simulink model "drone_simul10"  (R2022b)
settings: Solver=VariableStepAuto  StartTime=0.0  StopTime=10  RelTol=1e-3
model workspace (MAT data in the model file):
  Pmax = Simulink.Parameter
  Pmax.Value = 2
  Pmax.DataType = 'auto'
  Pmax.Complexity = 'real'
  Pmax.Dimensions = [1 1]
  g = Simulink.Parameter
  g.Value = 9.81
  g.DataType = 'auto'
  g.Complexity = 'real'
  g.Dimensions = [1 1]
libraries: slpidlib x4, aerolibanimutils x2
settings Model: Creator=Raphael  LastModifiedBy=Raphael
settings OptimizationCC: DefaultParameterBehavior=Inlined  UseDivisionForNetSlopeComputation=on  GainParamInheritBuiltInType=on  UseFloatMulNetSlope=on  InlineInvariantSignals=on  EnhancedBackFolding=on  BooleansAsBitfields=on  PassReuseOutputArgsAs=Individual arguments  StateBitsets=on  DataBitsets=on  ZeroExternalMemoryAtStartup=off  ZeroInternalMemoryAtStartup=off  NoFixptDivByZeroProtection=on  EfficientFloat2IntCast=on  LifeSpan=1  OptimizeBlockOrder=speed  DifferentSizesBufferReuse=on  EfficientTunableParamExpr=on
settings DebuggingCC: ParameterTunabilityLossMsg=error
settings HardwareCC: ProdBitPerLong=64  ProdHWDeviceType=AMD->x86-64 (Linux 64)
settings SFSimCC: MATLABDynamicMemAlloc=off
settings RTWCC: Description=Embedded Coder  SystemTargetFile=ert.tlc  GenCodeOnly=on  TemplateMakefile=ert_default_tmf
settings CodeAppCC: ForceParamTrailComments=on  IgnoreCustomStorageClasses=off  OperatorAnnotations=on  SimulinkDataObjDesc=on  SFDataObjDesc=on  CustomSymbolStrGlobalVar=rt$N$M  CustomSymbolStrType=$N$M  CustomSymbolStrFcn=$N$M$F  CustomSymbolStrMacro=$N$M  InsertBlockDesc=on
settings ERTTargetCC: TargetLangStandard=C99 (ISO)  GenerateSampleERTMain=on  IncludeMdlTerminateFcn=off  CombineSignalStateStructs=on  SupportAbsoluteTime=off  SupportComplex=off  SupportNonInlinedSFcns=on  InlinedParameterPlacement=NonHierarchical  ERTCustomFileTemplate=example_file_process.tlc  ERTFilePackagingFormat=CompactWithDataFile

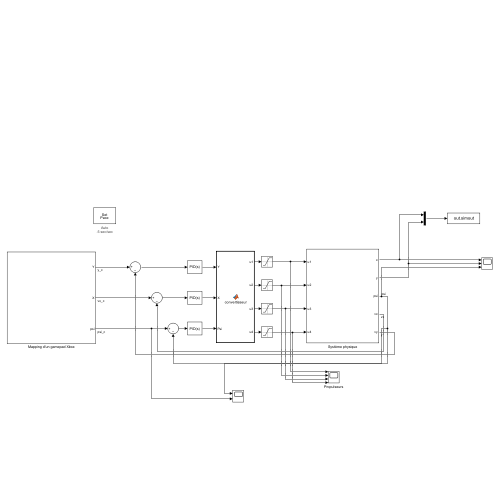
[thumbnail: Simulink's stored preview of the top-level diagram]
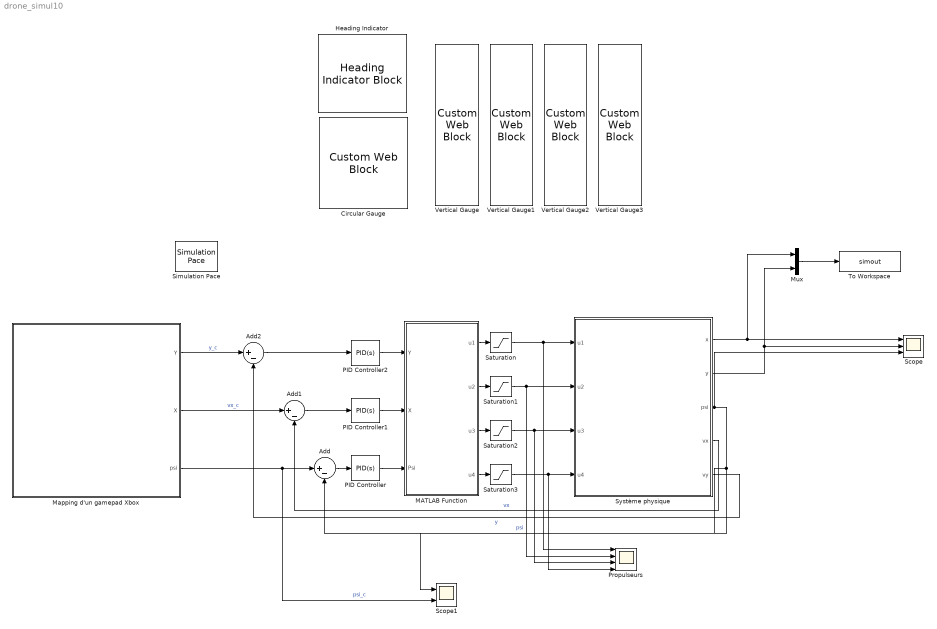
== system drone_simul10 ==
  Add : Sum  Inputs=|+-
  Add1 : Sum  Inputs=|+-
  Add2 : Sum  Inputs=|+-
  Circular Gauge : CustomWebBlock  LabelPosition=Hide  ShowInitialText=on  Configuration="{\"type\":\"CircularGauge\",\"settings\":{\"BindingType\":\"signal\",\"aspectRatio\":1.032258064516129,\"backgroundColor\":[0,0,0,\"1\"],\"backgroundOffset\":1,\"backgroundOpacity\":1,\"direction\":\"cw\",\"fixedAspectRatio\":\"on\",\"flipLimits\":0,\"orientation\":\"horizontal\",\"showBackgroundColor\":false,\"value\":0},\"components\":[{\"name\":\"CircularScaleComponent\",\"settings\":{\"bounds\":{\"max\":10,\"min\":-10,\"tickInterval\":\"auto\"},\"direction\":\"cw\",\"flipLimits\":0,\"innerRadius\":0.75,\"internalTickHeightScaleFactor\":1,\"labelColor\":[255,255,200],\"labelFont\":{\"font\":\"Arial\",\"fontSize\":12},\"labelRadius\":0.528,\"labelTransparency\":1,\"minorTickHeightScaleFactor\":0.2,\"needleImage\":{\"size\":[200,50],\"src\":\"data:image/svg+xml;base64,PD94bWwgdmVyc2lvbj0iMS4wIiBlbmNvZGluZz0idXRmLTgiPz4KPCEtLSBHZW5lcmF0b3I6IEFkb2JlIElsbHVzdHJhdG9yIDI0LjEuMiwgU1ZHIEV4cG9ydCBQbHVnLUluIC4gU1ZHIFZlcnNpb246IDYuMDAgQnVpbGQgMCkgIC0tPgo8c3ZnIHZlcnNpb249IjEuMSIgaWQ9IkxheWVyXzEiIHhtbG5zPSJodHRwOi8vd3d3LnczLm9yZy8yMDAwL3N2ZyIgeG1sbnM6eGxpbms9Imh0dHA6Ly93d3cudzMub3JnLzE5OTkveGxpbmsiIHg9IjBweCIgeT0iMHB4IgoJIHZpZXdCb3g9IjAgMCAyMDAgNTAiIHN0eWxlPSJlbmFibGUtYmFja2dyb3VuZDpuZXcgMCAwIDIwMCA1MDsiIHhtbDpzcGFjZT0icHJlc2VydmUiPgo8c3R5bGUgdHlwZT0idGV4dC9jc3MiPgoJLnN0MHtmaWxsOiNFQzIxMjc7fQo8L3N0eWxlPgo8cGF0aCBjbGFzcz0ic3QwIiBkPSJNMTYyLjgsMTMuN0MxNjksNC40LDE4MS43LDEuOSwxOTEsOC4xczExLjgsMTguOSw1LjYsMjguMnMtMTguOSwxMS44LTI4LjIsNS42bDAsMAoJQzE1OS4xLDM1LjYsMTU2LjYsMjMsMTYyLjgsMTMuN0wxNjIuOCwxMy43eiBNMTY1LjgsMTUuOGMtNS4xLDcuNi0zLjEsMTcuOSw0LjYsMjNjNy42LDUuMSwxNy45LDMuMSwyMy00LjYKCWM1LjEtNy42LDMuMS0xNy45LTQuNi0yM2wwLDBDMTgxLjIsNi4yLDE3MC45LDguMiwxNjUuOCwxNS44eiIvPgo8cGF0aCBjbGFzcz0ic3QwIiBkPSJNMC40LDI1Ljl2LTMuM2wxNTktMi41Yy0wLjcsMi42LTAuNyw1LjIsMCw3LjhMMC40LDI1Ljl6Ii8+CjxjaXJjbGUgY2xhc3M9InN0MCIgY3g9IjE3OS42IiBjeT0iMjQiIHI9IjAuNyIvPgo8L3N2Zz4K\"},\"needleOffset\":[0.18464878250906522,0],\"needleOrientation\":-45,\"needleRotation\":180,\"needleSize\":{\"height\":0.11741692305346914,\"width\":0.46108337545091255},\"outerRadius\":0.9,\"position\":[0.05,0.05,0.9,0.9],\"referencePoint\":\"auto\",\"scaleAngle\":270,\"scaleAngleOffset\":135,\"scaleColors\":[],\"scaleColorsSize\":0.2,\"scaleDirection\":\"CW\",\"scalePosition\":[0,0,1,1],\"showLabels\":1,\"showMinorTicks\":1,\"showSpanLine\":1,\"showTicks\":1,\"tickColor\":[252,252,197],\"tickTransparency\":1,\"valueBarColor\":[0,114,189],\"valueBarPosition\":[0,0,1,1],\"valueBarSize\":0.2,\"valueBarTransparency\":1}},{\"name\":\"BackgroundImageComponent\",\"settings\":{\"image\":{\"size\":[500,500],\"src\":\"data:image/svg+xml;base64,PD94bWwgdmVyc2lvbj0iMS4wIiBlbmNvZGluZz0iVVRGLTgiIHN0YW5kYWxvbmU9Im5vIj8+CjxzdmcKICAgeG1sbnM6ZGM9Imh0dHA6Ly9wdXJsLm9yZy9kYy9lbGVtZW50cy8xLjEvIgogICB4bWxuczpjYz0iaHR0cDovL2NyZWF0aXZlY29tbW9ucy5vcmcvbnMjIgogICB4bWxuczpyZGY9Imh0dHA6Ly93d3cudzMub3JnLzE5OTkvMDIvMjItcmRmLXN5bnRheC1ucyMiCiAgIHhtbG5zOnN2Zz0iaHR0cDovL3d3dy53My5vcmcvMjAwMC9zdmciCiAgIHhtbG5zPSJodHRwOi8vd3d3LnczLm9yZy8yMDAwL3N2ZyIKICAgeG1sbnM6 ...(+9964 chars)\"},\"position\":[0,0,1,1],\"scaleMode\":\"0\"}},{\"name\":\"ForegroundImageComponent\",\"settings\":{\"image\":{\"size\":[0,0],\"src\":\"default\",\"srcOrientation\":[]},\"isForeground\":1,\"position\":[0,0,1,1],\"scaleMode\":\"0\"}}]}"
  Heading Indicator : HeadingIndicatorBlock
  MATLAB Function : MATLAB Function  TreatAsAtomicUnit=on
  Mapping d'un gamepad Xbox : Subsystem
  Mux : Mux  Inputs=2
  PID Controller : slpidlib/PID Controller  Controller=PID  Form=Ideal  TimeDomain=Continuous-time  UseExternalTs=off  SampleTime=-1  IntegratorMethod=Forward Euler  FilterMethod=Forward Euler  ControllerParametersSource=internal  P=5  I=0  UseKiTs=off  D=0.04  N=100  UseFilter=on  TunerSelectOption=Transfer Function Based (PID Tuner App)  InitialConditionSource=internal  InitialConditionForIntegrator=0  InitialConditionForFilter=0  DifferentiatorICPrevScaledInput=0  ExternalReset=none  TrackingMode=off  Kt=1  LimitOutput=off  SatLimitsSource=internal  UpperSaturationLimit=inf  LowerSaturationLimit=-inf  LinearizeAsGain=on  AntiWindupMode=none  Kb=1  LimitIntegrator=off  UpperIntegratorSaturationLimit=inf  LowerIntegratorSaturationLimit=-inf  POutMin=[]  POutMax=[]  IOutMin=[]  IOutMax=[]  DOutMin=[]  DOutMax=[]  NOutMin=[]  NOutMax=[]  SumOutMin=[]  SumOutMax=[]  SaturationOutMin=[]  SaturationOutMax=[]  PParamMin=[]  PParamMax=[]  IParamMin=[]  IParamMax=[]  DParamMin=[]  DParamMax=[]  NParamMin=[]  NParamMax=[]  KbParamMin=[]  KbParamMax=[]  KtParamMin=[]  KtParamMax=[]  KbOutMin=[]  KbOutMax=[]  KtOutMin=[]  KtOutMax=[]  IntegratorOutMin=[]  IntegratorOutMax=[]  FilterOutMin=[]  FilterOutMax=[]  SumI1OutMin=[]  SumI1OutMax=[]  SumI2OutMin=[]  SumI2OutMax=[]  SumI3OutMin=[]  SumI3OutMax=[]  SumI4OutMin=[]  SumI4OutMax=[]  SumDOutMin=[]  SumDOutMax=[]  DifferentiatorOutMin=[]  DifferentiatorOutMax=[]  FilterDiffOutCoefMin=[]  FilterDiffOutCoefMax=[]  ReciprocalOutMin=[]  ReciprocalOutMax=[]  SumDenOutMin=[]  SumDenOutMax=[]  SumNumOutMin=[]  SumNumOutMax=[]  DivideOutMin=[]  DivideOutMax=[]  UdiffTsProdOutMin=[]  UdiffTsProdOutMax=[]  NTsProdOutMin=[]  NTsProdOutMax=[]  UintegralTsProdOutMin=[]  UintegralTsProdOutMax=[]  UngainTsProdOutMin=[]  UngainTsProdOutMax=[]  ClampingZeroOutDataTypeStr=Inherit: Inherit via back propagation  ClampingZeroOutMin=[]  ClampingZeroOutMax=[]  FilterDenConstantOutDataTypeStr=Inherit: Inherit via back propagation  FilterDenConstantOutMin=[]  FilterDenConstantOutMax=[]  PCopyOutDataTypeStr=Inherit: Inherit via back propagation  PCopyOutMin=[]  PCopyOutMax=[]  NCopyOutDataTypeStr=Inherit: Inherit via back propagation  NCopyOutMin=[]  NCopyOutMax=[]  IntegratorContinuousStateAttributes=''  IntegratorStateMustResolveToSignalObject=off  IntegratorRTWStateStorageClass=Auto  FilterContinuousStateAttributes=''  FilterStateMustResolveToSignalObject=off  FilterRTWStateStorageClass=Auto  ParallelPVariant=Passthrough  IdealPVariant=InternalParameters  IVariant=InternalParameters  DVariant=InternalParameters  IntegratorVariant=Continuous  SatVariant=Disabled  AWVariant=Passthrough  PCopyVariant=Disabled  TRVariant=Disabled  FdbkBlocksVariant=Forward  IdealPFdbkVariant=Disabled  SatFdbkVariant=Disabled  DerivativeFilterVariant=ContFilter  NVariant=InternalParameters  NCopyVariant=Disabled  FilterICVariant=InternalICsFilter  IntegratorICVariant=InternalICs  ExternalResetVariant=Disabled  TRSumVariant=Passthrough  SumFdbkVariant=Disabled  SumVariant=Sum_PID  TsampFilterVariant=InternalTs  TsampNgainVariant=Passthrough  TsampIntegralVariant=Passthrough  ExternalSaturationOutDataTypeStr=Inherit: Same as second input
  PID Controller1 : slpidlib/PID Controller  Controller=PID  Form=Ideal  TimeDomain=Continuous-time  UseExternalTs=off  SampleTime=-1  IntegratorMethod=Forward Euler  FilterMethod=Forward Euler  ControllerParametersSource=internal  P=5  I=0.1  UseKiTs=off  D=0  N=100  UseFilter=on  TunerSelectOption=Transfer Function Based (PID Tuner App)  InitialConditionSource=internal  InitialConditionForIntegrator=0  InitialConditionForFilter=0  DifferentiatorICPrevScaledInput=0  ExternalReset=none  TrackingMode=off  Kt=1  LimitOutput=off  SatLimitsSource=internal  UpperSaturationLimit=inf  LowerSaturationLimit=-inf  LinearizeAsGain=on  AntiWindupMode=none  Kb=1  LimitIntegrator=off  UpperIntegratorSaturationLimit=inf  LowerIntegratorSaturationLimit=-inf  POutMin=[]  POutMax=[]  IOutMin=[]  IOutMax=[]  DOutMin=[]  DOutMax=[]  NOutMin=[]  NOutMax=[]  SumOutMin=[]  SumOutMax=[]  SaturationOutMin=[]  SaturationOutMax=[]  PParamMin=[]  PParamMax=[]  IParamMin=[]  IParamMax=[]  DParamMin=[]  DParamMax=[]  NParamMin=[]  NParamMax=[]  KbParamMin=[]  KbParamMax=[]  KtParamMin=[]  KtParamMax=[]  KbOutMin=[]  KbOutMax=[]  KtOutMin=[]  KtOutMax=[]  IntegratorOutMin=[]  IntegratorOutMax=[]  FilterOutMin=[]  FilterOutMax=[]  SumI1OutMin=[]  SumI1OutMax=[]  SumI2OutMin=[]  SumI2OutMax=[]  SumI3OutMin=[]  SumI3OutMax=[]  SumI4OutMin=[]  SumI4OutMax=[]  SumDOutMin=[]  SumDOutMax=[]  DifferentiatorOutMin=[]  DifferentiatorOutMax=[]  FilterDiffOutCoefMin=[]  FilterDiffOutCoefMax=[]  ReciprocalOutMin=[]  ReciprocalOutMax=[]  SumDenOutMin=[]  SumDenOutMax=[]  SumNumOutMin=[]  SumNumOutMax=[]  DivideOutMin=[]  DivideOutMax=[]  UdiffTsProdOutMin=[]  UdiffTsProdOutMax=[]  NTsProdOutMin=[]  NTsProdOutMax=[]  UintegralTsProdOutMin=[]  UintegralTsProdOutMax=[]  UngainTsProdOutMin=[]  UngainTsProdOutMax=[]  ClampingZeroOutDataTypeStr=Inherit: Inherit via back propagation  ClampingZeroOutMin=[]  ClampingZeroOutMax=[]  FilterDenConstantOutDataTypeStr=Inherit: Inherit via back propagation  FilterDenConstantOutMin=[]  FilterDenConstantOutMax=[]  PCopyOutDataTypeStr=Inherit: Inherit via back propagation  PCopyOutMin=[]  PCopyOutMax=[]  NCopyOutDataTypeStr=Inherit: Inherit via back propagation  NCopyOutMin=[]  NCopyOutMax=[]  IntegratorContinuousStateAttributes=''  IntegratorStateMustResolveToSignalObject=off  IntegratorRTWStateStorageClass=Auto  FilterContinuousStateAttributes=''  FilterStateMustResolveToSignalObject=off  FilterRTWStateStorageClass=Auto  ParallelPVariant=Passthrough  IdealPVariant=InternalParameters  IVariant=InternalParameters  DVariant=InternalParameters  IntegratorVariant=Continuous  SatVariant=Disabled  AWVariant=Passthrough  PCopyVariant=Disabled  TRVariant=Disabled  FdbkBlocksVariant=Forward  IdealPFdbkVariant=Disabled  SatFdbkVariant=Disabled  DerivativeFilterVariant=ContFilter  NVariant=InternalParameters  NCopyVariant=Disabled  FilterICVariant=InternalICsFilter  IntegratorICVariant=InternalICs  ExternalResetVariant=Disabled  TRSumVariant=Passthrough  SumFdbkVariant=Disabled  SumVariant=Sum_PID  TsampFilterVariant=InternalTs  TsampNgainVariant=Passthrough  TsampIntegralVariant=Passthrough  ExternalSaturationOutDataTypeStr=Inherit: Same as second input
  PID Controller2 : slpidlib/PID Controller  Controller=PID  Form=Ideal  TimeDomain=Continuous-time  UseExternalTs=off  SampleTime=-1  IntegratorMethod=Forward Euler  FilterMethod=Forward Euler  ControllerParametersSource=internal  P=5  I=0  UseKiTs=off  D=0.3  N=100  UseFilter=on  TunerSelectOption=Transfer Function Based (PID Tuner App)  InitialConditionSource=internal  InitialConditionForIntegrator=0  InitialConditionForFilter=0  DifferentiatorICPrevScaledInput=0  ExternalReset=none  TrackingMode=off  Kt=1  LimitOutput=off  SatLimitsSource=internal  UpperSaturationLimit=inf  LowerSaturationLimit=-inf  LinearizeAsGain=on  AntiWindupMode=none  Kb=1  LimitIntegrator=off  UpperIntegratorSaturationLimit=inf  LowerIntegratorSaturationLimit=-inf  POutMin=[]  POutMax=[]  IOutMin=[]  IOutMax=[]  DOutMin=[]  DOutMax=[]  NOutMin=[]  NOutMax=[]  SumOutMin=[]  SumOutMax=[]  SaturationOutMin=[]  SaturationOutMax=[]  PParamMin=[]  PParamMax=[]  IParamMin=[]  IParamMax=[]  DParamMin=[]  DParamMax=[]  NParamMin=[]  NParamMax=[]  KbParamMin=[]  KbParamMax=[]  KtParamMin=[]  KtParamMax=[]  KbOutMin=[]  KbOutMax=[]  KtOutMin=[]  KtOutMax=[]  IntegratorOutMin=[]  IntegratorOutMax=[]  FilterOutMin=[]  FilterOutMax=[]  SumI1OutMin=[]  SumI1OutMax=[]  SumI2OutMin=[]  SumI2OutMax=[]  SumI3OutMin=[]  SumI3OutMax=[]  SumI4OutMin=[]  SumI4OutMax=[]  SumDOutMin=[]  SumDOutMax=[]  DifferentiatorOutMin=[]  DifferentiatorOutMax=[]  FilterDiffOutCoefMin=[]  FilterDiffOutCoefMax=[]  ReciprocalOutMin=[]  ReciprocalOutMax=[]  SumDenOutMin=[]  SumDenOutMax=[]  SumNumOutMin=[]  SumNumOutMax=[]  DivideOutMin=[]  DivideOutMax=[]  UdiffTsProdOutMin=[]  UdiffTsProdOutMax=[]  NTsProdOutMin=[]  NTsProdOutMax=[]  UintegralTsProdOutMin=[]  UintegralTsProdOutMax=[]  UngainTsProdOutMin=[]  UngainTsProdOutMax=[]  ClampingZeroOutDataTypeStr=Inherit: Inherit via back propagation  ClampingZeroOutMin=[]  ClampingZeroOutMax=[]  FilterDenConstantOutDataTypeStr=Inherit: Inherit via back propagation  FilterDenConstantOutMin=[]  FilterDenConstantOutMax=[]  PCopyOutDataTypeStr=Inherit: Inherit via back propagation  PCopyOutMin=[]  PCopyOutMax=[]  NCopyOutDataTypeStr=Inherit: Inherit via back propagation  NCopyOutMin=[]  NCopyOutMax=[]  IntegratorContinuousStateAttributes=''  IntegratorStateMustResolveToSignalObject=off  IntegratorRTWStateStorageClass=Auto  FilterContinuousStateAttributes=''  FilterStateMustResolveToSignalObject=off  FilterRTWStateStorageClass=Auto  ParallelPVariant=Passthrough  IdealPVariant=InternalParameters  IVariant=InternalParameters  DVariant=InternalParameters  IntegratorVariant=Continuous  SatVariant=Disabled  AWVariant=Passthrough  PCopyVariant=Disabled  TRVariant=Disabled  FdbkBlocksVariant=Forward  IdealPFdbkVariant=Disabled  SatFdbkVariant=Disabled  DerivativeFilterVariant=ContFilter  NVariant=InternalParameters  NCopyVariant=Disabled  FilterICVariant=InternalICsFilter  IntegratorICVariant=InternalICs  ExternalResetVariant=Disabled  TRSumVariant=Passthrough  SumFdbkVariant=Disabled  SumVariant=Sum_PID  TsampFilterVariant=InternalTs  TsampNgainVariant=Passthrough  TsampIntegralVariant=Passthrough  ExternalSaturationOutDataTypeStr=Inherit: Same as second input
  Propulseurs : Scope  NumInputPorts=4
  Saturation{,1..3} (4 alike) : Saturate  UpperLimit=Pmax*g  LowerLimit=0
  Scope : Scope  NumInputPorts=3
  Scope1 : Scope  NumInputPorts=2
  Simulation Pace : aerolibanimutils/Simulation Pace  SimulationPace=.5  SleepMode=Auto  OutputPaceError=off  SampleTime=1/30
  Système physique : Subsystem
  To Workspace : ToWorkspace  VariableName=simout  SaveFormat=Timeseries  SampleTime=-1
  Vertical Gauge{,1..3} (4 alike) : CustomWebBlock  LabelPosition=Hide  ShowInitialText=on  Configuration="{\"type\":\"LinearGauge\",\"settings\":{\"BindingType\":\"signal\",\"backgroundColor\":[0,0,0,\"1\"],\"backgroundOffset\":0,\"backgroundOpacity\":1,\"fixedAspectRatio\":\"on\",\"orientation\":\"vertical\",\"showBackgroundColor\":false,\"value\":0},\"components\":[{\"name\":\"LinearScaleComponent\",\"settings\":{\"bounds\":{\"max\":20,\"min\":0,\"tickInterval\":\"auto\"},\"internalTickHeightScaleFactor\":0.5,\"labelColor\":[255,255,200],\"labelFont\":{\"font\":\"Arial\",\"fontSize\":12},\"labelOffset\":0.05,\"labelTransparency\":1,\"needleImage\":{\"size\":[21,75],\"src\":\"data:image/svg+xml;base64,PHN2ZyB4bWxucz0iaHR0cDovL3d3dy53My5vcmcvMjAwMC9zdmciIHhtbG5zOnhsaW5rPSJodHRwOi8vd3d3LnczLm9yZy8xOTk5L3hsaW5rIiB2aWV3Qm94PSIwIDAgMjEgNzUiPjxkZWZzPjxzdHlsZT4uY2xzLTF7ZmlsbDpub25lO30uY2xzLTJ7aXNvbGF0aW9uOmlzb2xhdGU7fS5jbHMtM3tjbGlwLXBhdGg6dXJsKCNjbGlwLXBhdGgpO30uY2xzLTR7b3BhY2l0eTowLjM7bWl4LWJsZW5kLW1vZGU6bXVsdGlwbHk7fS5jbHMtNXtmaWxsOiNlYjI2Mjk7fTwvc3R5bGU+PGNsaXBQYXRoIGlkPSJjbGlwLXBhdGgiIHRyYW5zZm9y ...(+1928 chars)\",\"srcOrientation\":\"horizontal\"},\"needleOffset\":[0.007413509060955519,0],\"needleSize\":{\"height\":0.11955094537815127,\"width\":0.7589285714285714},\"position\":[0.015821953781512604,0.06944444444444445,0.7996031746031746,0.9641544117647058],\"referencePoint\":\"auto\",\"scaleColors\":[{\"Color\":[254,51,10],\"Max\":20,\"Min\":18}],\"scaleColorsSize\":0.2,\"scaleDirection\":\"BT\",\"showLabels\":1,\"showMinorTicks\":0,\"showSpanLine\":1,\"showTicks\":1,\"tickColor\":[252,252,197],\"tickTransparency\":1,\"valueBarColor\":[23,89,176],\"valueBarOffset\":0,\"valueBarSize\":0.23,\"valueBarTransparency\":1}},{\"name\":\"BackgroundImageComponent\",\"settings\":{\"image\":{\"size\":[380,101],\"src\":\"data:image/svg+xml;base64,PHN2ZyBpZD0iZnJhbWUiIHhtbG5zPSJodHRwOi8vd3d3LnczLm9yZy8yMDAwL3N2ZyIgeG1sbnM6eGxpbms9Imh0dHA6Ly93d3cudzMub3JnLzE5OTkveGxpbmsiIHZpZXdCb3g9IjAgMCAzODAgMTAxIj48ZGVmcz48c3R5bGU+LmNscy0xe2ZpbGw6IzAwMmI0Mjt9LmNscy0ye2ZpbGw6IzQyNzA4Mjt9LmNscy0ze2ZpbGw6dXJsKCNyYWRpYWwtZ3JhZGllbnQpO308L3N0eWxlPjxyYWRpYWxHcmFkaWVudCBpZD0icmFkaWFsLWdyYWRpZW50IiBjeD0iMTkwIiBjeT0iNTAuNSIgcj0iMjY5LjIxIiBncmFkaWVudFVuaXRzPSJ1c2VyU3BhY2VPblVzZSI+PHN0b3Agb2Zmc2V0PSIwLjAxIiBzdG9wLWNvbG9yPSIjM2U0ZjU4Ii8+PHN0b3Agb2Zmc2V0PSIwLjA2IiBzdG9wLWNvbG9yPSIjNDQ1NzYxIi8+PHN0b3Agb2Zmc2V0PSIwLjE1IiBzdG9wLWNvbG9yPSIjNTU2YTc2Ii8+PHN0b3Agb2Zmc2V0PSIwLjI1IiBzdG9wLWNvbG9yPSIjNmQ4ODk1Ii8+PHN0b3Agb2Zmc2V0PSIwLjM4IiBzdG9wLWNvbG9yPSIjOGZiMmMzIi8+PHN0b3Agb2Zmc2V0PSIwLjUyIiBzdG9wLWNvbG9yPSIjYjZlNGZhIi8+PHN0b3Agb2Zmc2V0PSIxIiBzdG9wLWNvbG9yPSIjMTU0NjU3Ii8+PC9yYWRpYWxHcmFkaWVudD48L2RlZnM+PGcgaWQ9IkxheWVyXzIiIGRhdGEtbmFtZT0iTGF5ZXIgMiI+PGcgaWQ9IkxheWVyXzEtMiIgZGF0YS1uYW1lPSJMYXllciAxLTIiPjxyZWN0IGlkPSJyZWN0MTAzNiIgY2xhc3M9ImNscy0xIiB4PSIxMSIgeT0iMTEiIHdpZHRoPSIzNTgiIGhlaWdodD0iNzkiLz48cGF0aCBpZD0icGF0aDEwMzgiIGNsYXNzPSJjbHMtMiIgZD0iTTgsOFY5M0gzNzJWOFpNMzY5LDkwSDExVjExSDM2OVoiLz48cGF0aCBpZD0icGF0aDEwNDAiIGNsYXNzPSJjbHMtMyIgZD0iTTAsMFYxMDFIMzgwVjBaTTM3Miw5M0g4VjhIMzcyWiIvPjwvZz48L2c+PC9zdmc+\",\"srcOrientation\":\"horizontal\"},\"position\":[0,0,1,1],\"scaleMode\":\"0\"}},{\"name\":\"ForegroundImageComponent\",\"settings\":{\"image\":{\"size\":[0,0],\"src\":\"default\",\"srcOrientation\":[]},\"isForeground\":1,\"position\":[0,0,1,1],\"scaleMode\":\"0\"}}]}"
  wires:
  Système physique/2(y) -> Scope/2, Mux/2
  Système physique/1(x) -> Scope/1, Mux/1
  Système physique/3(psi) -> Scope/3, Scope1/1, Add/2  "psi"
  MATLAB Function/1(u1) -> Saturation/1
  MATLAB Function/2(u2) -> Saturation1/1
  MATLAB Function/3(u3) -> Saturation2/1
  MATLAB Function/4(u4) -> Saturation3/1
  Mux/1 -> To Workspace/1
  Add/1 -> PID Controller/1
  Système physique/4(vx) -> Add1/2  "vx"
  Add1/1 -> PID Controller1/1
  Saturation/1 -> Propulseurs/1, Système physique/1(u1)
  Saturation1/1 -> Propulseurs/2, Système physique/2(u2)
  Saturation2/1 -> Propulseurs/3, Système physique/3(u3)
  Saturation3/1 -> Propulseurs/4, Système physique/4(u4)
  Système physique/5(vy) -> Add2/2  "y"
  Mapping d'un gamepad Xbox/1(Y) -> Add2/1  "y_c"
  Add2/1 -> PID Controller2/1
  Mapping d'un gamepad Xbox/2(X) -> Add1/1  "vx_c"
  Mapping d'un gamepad Xbox/3(psi) -> Scope1/2, Add/1  "psi_c"
  PID Controller/1 -> MATLAB Function/3(Psi)
  PID Controller2/1 -> MATLAB Function/1(Y)
  PID Controller1/1 -> MATLAB Function/2(X)

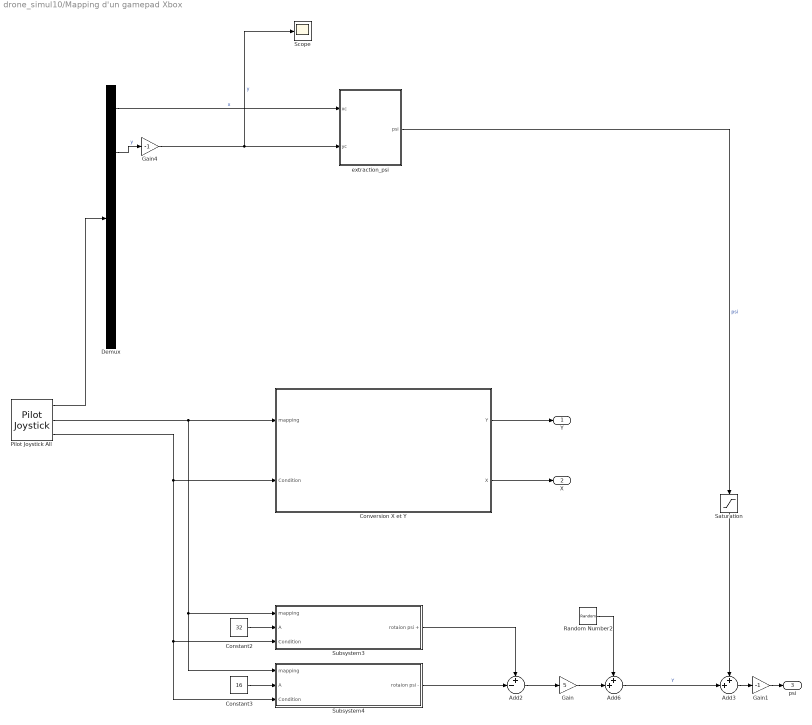
== system drone_simul10/Mapping d'un gamepad Xbox ==
  Add2 : Sum  Inputs=+-|
  Add3 : Sum  Inputs=++|
  Add6 : Sum  Inputs=++|
  Constant2 : Constant  Value=32
  Constant3 : Constant  Value=16
  Conversion X et Y : Subsystem
  Demux : Demux  Outputs=6
  Gain : Gain  Gain=5
  Gain1 : Gain  Gain=-1
  Gain4 : Gain  Gain=-1
  Pilot Joystick All : aerolibanimutils/Pilot Joystick  JoystickID=Joystick2  OutputConfiguration=AllOutputs  SampleTime=0.01
      settings: LibrarySourceBlock=aerolibanimutils/Pilot Joystick All
  Random Number2 : RandomNumber  Variance=0.002  Seed=12  SampleTime=0.1
  Saturation : Saturate  UpperLimit=45  LowerLimit=-45
  Scope : Scope
  Subsystem3 : Subsystem
  Subsystem4 : Subsystem
  extraction_psi : MATLAB Function  TreatAsAtomicUnit=on
  Y : Outport
  X : Outport  Port=2
  psi : Outport  Port=3
  wires:
  Pilot Joystick All/1 -> Demux/1
  Gain4/1 -> Scope/1, extraction_psi/2(yc)  "y"
  Demux/2 -> Gain4/1  "y"
  Demux/1 -> extraction_psi/1(xc)  "x"
  Pilot Joystick All/3 -> Subsystem4/3(Condition), Subsystem3/3(Condition), Conversion X et Y/2(Condition)
  Pilot Joystick All/2 -> Conversion X et Y/1(mapping), Subsystem4/1(mapping), Subsystem3/1(mapping)
  Constant2/1 -> Subsystem3/2(A)
  Constant3/1 -> Subsystem4/2(A)
  Subsystem4/1(rotaion psi -) -> Add2/2
  Subsystem3/1(rotaion psi +) -> Add2/1
  Add3/1 -> Gain1/1
  Add2/1 -> Gain/1
  Saturation/1 -> Add3/1
  extraction_psi/1(psi) -> Saturation/1  "psi"
  Conversion X et Y/1(Y) -> Y/1
  Conversion X et Y/2(X) -> X/1
  Gain1/1 -> psi/1
  Gain/1 -> Add6/2
  Random Number2/1 -> Add6/1
  Add6/1 -> Add3/2  "Y"

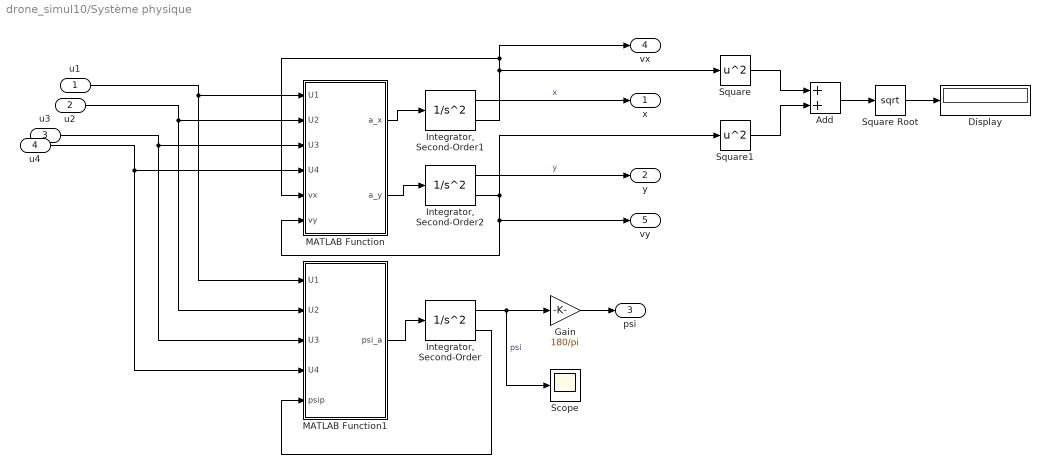
== system drone_simul10/Système physique ==
  u1 : Inport
  u2 : Inport  Port=2
  u3 : Inport  Port=3
  u4 : Inport  Port=4
  Add : Sum
  Display : Display
  Gain : Gain  Gain=180/pi
  "Integrator, Second-Order" : SecondOrderIntegrator
  "Integrator, Second-Order1" : SecondOrderIntegrator  ICX=0
  "Integrator, Second-Order2" : SecondOrderIntegrator  ICX=0
  MATLAB Function : MATLAB Function  TreatAsAtomicUnit=on
  MATLAB Function1 : MATLAB Function  TreatAsAtomicUnit=on
  Scope : Scope
  Square : Math  Operator=square
  Square Root : Sqrt
  Square1 : Math  Operator=square
  x : Outport
  y : Outport  Port=2
  psi : Outport  Port=3
  vx : Outport  Port=4
  vy : Outport  Port=5
  wires:
  u4/1 -> MATLAB Function1/4(U4), MATLAB Function/4(U4)
  "Integrator, Second-Order1"/1 -> x/1  "x"
  u1/1 -> MATLAB Function1/1(U1), MATLAB Function/1(U1)
  "Integrator, Second-Order"/1 -> Scope/1, Gain/1  "psi"
  "Integrator, Second-Order1"/2 -> Square/1, vx/1, MATLAB Function/5(vx)
  "Integrator, Second-Order2"/2 -> vy/1, MATLAB Function/6(vy), Square1/1
  MATLAB Function1/1(psi_a) -> "Integrator, Second-Order"/1
  MATLAB Function/2(a_y) -> "Integrator, Second-Order2"/1
  u3/1 -> MATLAB Function/3(U3), MATLAB Function1/3(U3)
  MATLAB Function/1(a_x) -> "Integrator, Second-Order1"/1
  u2/1 -> MATLAB Function1/2(U2), MATLAB Function/2(U2)
  "Integrator, Second-Order2"/1 -> y/1  "y"
  "Integrator, Second-Order"/2 -> MATLAB Function1/5(psip)
  Gain/1 -> psi/1
  Square/1 -> Add/1
  Square1/1 -> Add/2
  Add/1 -> Square Root/1
  Square Root/1 -> Display/1

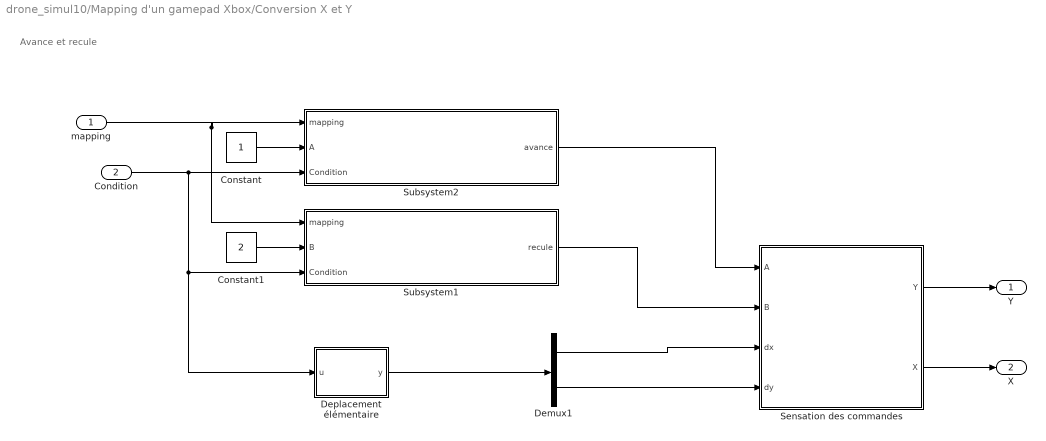
== system drone_simul10/Mapping d'un gamepad Xbox/Conversion X et Y ==
  note: Avance et recule
  mapping : Inport
  Condition : Inport  Port=2
  Constant : Constant
  Constant1 : Constant  Value=2
  Demux1 : Demux  Outputs=2
  Deplacement élémentaire : MATLAB Function  TreatAsAtomicUnit=on
  Sensation des commandes : Subsystem
  Subsystem1 : Subsystem
  Subsystem2 : Subsystem
  Y : Outport
  X : Outport  Port=2
  wires:
  Deplacement élémentaire/1(y) -> Demux1/1
  Constant1/1 -> Subsystem1/2(B)
  Condition/1 -> Deplacement élémentaire/1(u), Subsystem1/3(Condition), Subsystem2/3(Condition)
  Constant/1 -> Subsystem2/2(A)
  mapping/1 -> Subsystem1/1(mapping), Subsystem2/1(mapping)
  Subsystem2/1(avance) -> Sensation des commandes/1(A)
  Subsystem1/1(recule) -> Sensation des commandes/2(B)
  Demux1/1 -> Sensation des commandes/3(dx)
  Demux1/2 -> Sensation des commandes/4(dy)
  Sensation des commandes/1(Y) -> Y/1
  Sensation des commandes/2(X) -> X/1

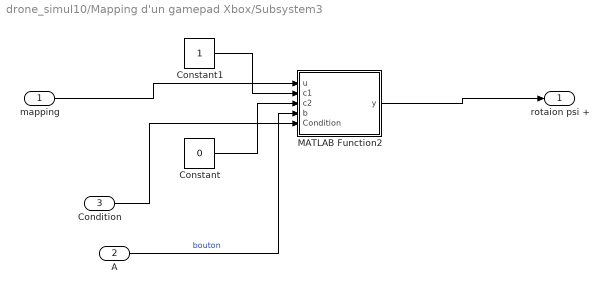
== system drone_simul10/Mapping d'un gamepad Xbox/Subsystem3 ==
  mapping : Inport
  A : Inport  Port=2
  Condition : Inport  Port=3
  Constant : Constant  Value=0
  Constant1 : Constant
  MATLAB Function2 : MATLAB Function  TreatAsAtomicUnit=on
  rotaion psi + : Outport
  wires:
  A/1 -> MATLAB Function2/4(b)  "bouton"
  mapping/1 -> MATLAB Function2/1(u)
  Constant1/1 -> MATLAB Function2/2(c1)
  Constant/1 -> MATLAB Function2/3(c2)
  MATLAB Function2/1(y) -> rotaion psi +/1
  Condition/1 -> MATLAB Function2/5(Condition)

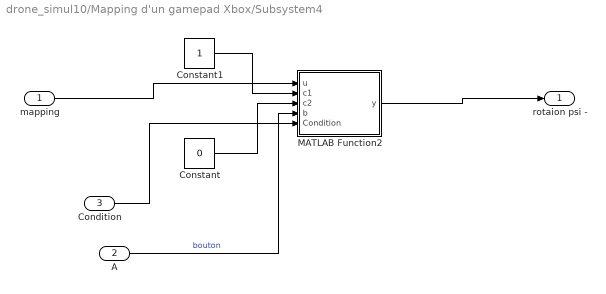
== system drone_simul10/Mapping d'un gamepad Xbox/Subsystem4 ==
  mapping : Inport
  A : Inport  Port=2
  Condition : Inport  Port=3
  Constant : Constant  Value=0
  Constant1 : Constant
  MATLAB Function2 : MATLAB Function  TreatAsAtomicUnit=on
  rotaion psi - : Outport
  wires:
  A/1 -> MATLAB Function2/4(b)  "bouton"
  mapping/1 -> MATLAB Function2/1(u)
  Constant1/1 -> MATLAB Function2/2(c1)
  Constant/1 -> MATLAB Function2/3(c2)
  MATLAB Function2/1(y) -> rotaion psi -/1
  Condition/1 -> MATLAB Function2/5(Condition)

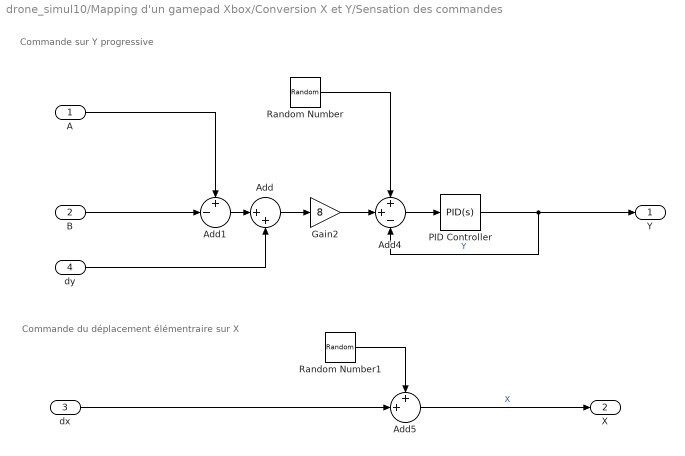
== system drone_simul10/Mapping d'un gamepad Xbox/Conversion X et Y/Sensation des commandes ==
  note: Commande du déplacement élémentraire sur X
  note: Commande sur Y progressive
  A : Inport
  B : Inport  Port=2
  dx : Inport  Port=3
  dy : Inport  Port=4
  Add : Sum  Inputs=|++
  Add1 : Sum  Inputs=+-|
  Add4 : Sum  Inputs=++-
  Add5 : Sum  Inputs=++|
  Gain2 : Gain  Gain=8
  PID Controller : slpidlib/PID Controller  Controller=PID  Form=Parallel  TimeDomain=Continuous-time  UseExternalTs=off  SampleTime=-1  IntegratorMethod=Forward Euler  FilterMethod=Forward Euler  ControllerParametersSource=internal  P=0  I=2.5  UseKiTs=off  D=0  N=100  UseFilter=on  TunerSelectOption=Transfer Function Based (PID Tuner App)  InitialConditionSource=internal  InitialConditionForIntegrator=0  InitialConditionForFilter=0  DifferentiatorICPrevScaledInput=0  ExternalReset=none  TrackingMode=off  Kt=1  LimitOutput=off  SatLimitsSource=internal  UpperSaturationLimit=inf  LowerSaturationLimit=-inf  LinearizeAsGain=on  AntiWindupMode=none  Kb=1  LimitIntegrator=off  UpperIntegratorSaturationLimit=inf  LowerIntegratorSaturationLimit=-inf  POutMin=[]  POutMax=[]  IOutMin=[]  IOutMax=[]  DOutMin=[]  DOutMax=[]  NOutMin=[]  NOutMax=[]  SumOutMin=[]  SumOutMax=[]  SaturationOutMin=[]  SaturationOutMax=[]  PParamMin=[]  PParamMax=[]  IParamMin=[]  IParamMax=[]  DParamMin=[]  DParamMax=[]  NParamMin=[]  NParamMax=[]  KbParamMin=[]  KbParamMax=[]  KtParamMin=[]  KtParamMax=[]  KbOutMin=[]  KbOutMax=[]  KtOutMin=[]  KtOutMax=[]  IntegratorOutMin=[]  IntegratorOutMax=[]  FilterOutMin=[]  FilterOutMax=[]  SumI1OutMin=[]  SumI1OutMax=[]  SumI2OutMin=[]  SumI2OutMax=[]  SumI3OutMin=[]  SumI3OutMax=[]  SumI4OutMin=[]  SumI4OutMax=[]  SumDOutMin=[]  SumDOutMax=[]  DifferentiatorOutMin=[]  DifferentiatorOutMax=[]  FilterDiffOutCoefMin=[]  FilterDiffOutCoefMax=[]  ReciprocalOutMin=[]  ReciprocalOutMax=[]  SumDenOutMin=[]  SumDenOutMax=[]  SumNumOutMin=[]  SumNumOutMax=[]  DivideOutMin=[]  DivideOutMax=[]  UdiffTsProdOutMin=[]  UdiffTsProdOutMax=[]  NTsProdOutMin=[]  NTsProdOutMax=[]  UintegralTsProdOutMin=[]  UintegralTsProdOutMax=[]  UngainTsProdOutMin=[]  UngainTsProdOutMax=[]  ClampingZeroOutDataTypeStr=Inherit: Inherit via back propagation  ClampingZeroOutMin=[]  ClampingZeroOutMax=[]  FilterDenConstantOutDataTypeStr=Inherit: Inherit via back propagation  FilterDenConstantOutMin=[]  FilterDenConstantOutMax=[]  PCopyOutDataTypeStr=Inherit: Inherit via back propagation  PCopyOutMin=[]  PCopyOutMax=[]  NCopyOutDataTypeStr=Inherit: Inherit via back propagation  NCopyOutMin=[]  NCopyOutMax=[]  IntegratorContinuousStateAttributes=''  IntegratorStateMustResolveToSignalObject=off  IntegratorRTWStateStorageClass=Auto  FilterContinuousStateAttributes=''  FilterStateMustResolveToSignalObject=off  FilterRTWStateStorageClass=Auto  ParallelPVariant=InternalParameters  IdealPVariant=Disabled  IVariant=InternalParameters  DVariant=InternalParameters  IntegratorVariant=Continuous  SatVariant=Disabled  AWVariant=Passthrough  PCopyVariant=Disabled  TRVariant=Disabled  FdbkBlocksVariant=Forward  IdealPFdbkVariant=Disabled  SatFdbkVariant=Disabled  DerivativeFilterVariant=ContFilter  NVariant=InternalParameters  NCopyVariant=Disabled  FilterICVariant=InternalICsFilter  IntegratorICVariant=InternalICs  ExternalResetVariant=Disabled  TRSumVariant=Passthrough  SumFdbkVariant=Disabled  SumVariant=Sum_PID  TsampFilterVariant=InternalTs  TsampNgainVariant=Passthrough  TsampIntegralVariant=Passthrough  ExternalSaturationOutDataTypeStr=Inherit: Same as second input
  Random Number : RandomNumber  Variance=0.002  SampleTime=0.1
  Random Number1 : RandomNumber  Variance=0.002  Seed=52  SampleTime=0.1
  Y : Outport
  X : Outport  Port=2
  wires:
  PID Controller/1 -> Y/1, Add4/3  "Y"
  Add5/1 -> X/1  "X"
  dx/1 -> Add5/2
  Add1/1 -> Add/1
  Add/1 -> Gain2/1
  Add4/1 -> PID Controller/1
  Gain2/1 -> Add4/2
  Random Number1/1 -> Add5/1
  Random Number/1 -> Add4/1
  A/1 -> Add1/1
  B/1 -> Add1/2
  dy/1 -> Add/2

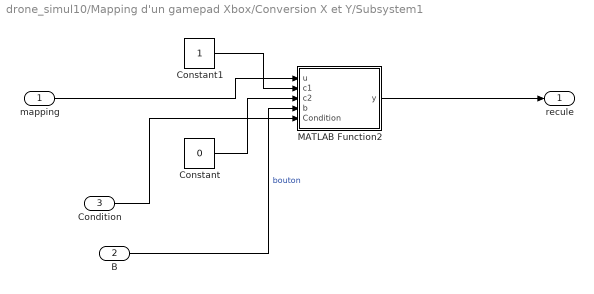
== system drone_simul10/Mapping d'un gamepad Xbox/Conversion X et Y/Subsystem1 ==
  mapping : Inport
  B : Inport  Port=2
  Condition : Inport  Port=3
  Constant : Constant  Value=0
  Constant1 : Constant
  MATLAB Function2 : MATLAB Function  TreatAsAtomicUnit=on
  recule : Outport
  wires:
  B/1 -> MATLAB Function2/4(b)  "bouton"
  mapping/1 -> MATLAB Function2/1(u)
  Constant1/1 -> MATLAB Function2/2(c1)
  Constant/1 -> MATLAB Function2/3(c2)
  MATLAB Function2/1(y) -> recule/1
  Condition/1 -> MATLAB Function2/5(Condition)

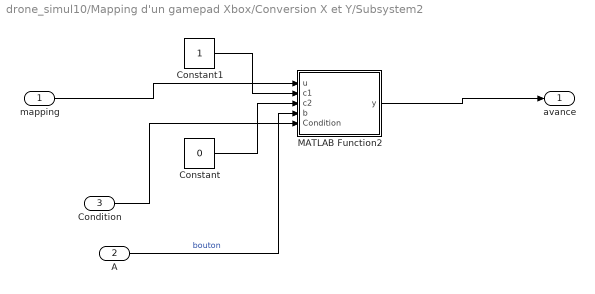
== system drone_simul10/Mapping d'un gamepad Xbox/Conversion X et Y/Subsystem2 ==
  mapping : Inport
  A : Inport  Port=2
  Condition : Inport  Port=3
  Constant : Constant  Value=0
  Constant1 : Constant
  MATLAB Function2 : MATLAB Function  TreatAsAtomicUnit=on
  avance : Outport
  wires:
  A/1 -> MATLAB Function2/4(b)  "bouton"
  mapping/1 -> MATLAB Function2/1(u)
  Constant1/1 -> MATLAB Function2/2(c1)
  Constant/1 -> MATLAB Function2/3(c2)
  MATLAB Function2/1(y) -> avance/1
  Condition/1 -> MATLAB Function2/5(Condition)

== matlab function drone_simul10/Mapping d'un gamepad Xbox/Subsystem4/MATLAB Function2 ==
  data: u input; y output; c1 input; c2 input; b input; Condition input
function y = cas(u, c1, c2, b, Condition)

if ((u == b) && (Condition==655.35))
    y = c1;
else
    y = c2;
end

== matlab function drone_simul10/Système physique/MATLAB Function1 ==
  data: U1 input; psi_a output; U2 input; U3 input; U4 input; psip input
function psi_a  = rotation(U1,U2,U3,U4,psip)

% Les constantes du bolides
m = 2;
l = 0.15;       % demi largeur du bolide
L = 0.30;       % demi longueur du bolide
K = 0.15;       % coefficient de frottement
Ioz = m/12*((2*l)^2+(2*L)^2);
% Construction des points

theta_or = pi/4;

psi_a = 1/Ioz*(-K*psip*L + L*sin(theta_or)*(-abs(U1)+abs(U2)-abs(U3)+abs(U4))+l*cos(theta_or)*(-abs(U1)+abs(U2)-abs(U3)+abs(U4)));

== matlab function drone_simul10/Système physique/MATLAB Function ==
  data: U1 input; a_x output; U2 input; U3 input; U4 input; vx input; vy input; a_y output
function [a_x, a_y] = translation(U1,U2,U3,U4,vx,vy)

% Les constantes du bolides
K = 0.15;       % coefficient de frottement
m = 2;
l = 0.15;       % demi largeur du bolide
L = 0.30;       % demi longueur du bolide

% Construction des points
theta_or = pi/4;


a_x = 1/m*(sin(theta_or)*(-abs(U1)+abs(U2)+abs(U3)-abs(U4))-K*vx);
a_y = 1/m*(cos(theta_or)*(abs(U1)+abs(U2)-abs(U3)-abs(U4))-K*vy);

== matlab function drone_simul10/Mapping d'un gamepad Xbox/extraction_psi ==
  data: xc input; psi output; yc input
function psi  = direction(xc,yc)

%% Fonction de conversion d'un joystick à un gamepad
if (sqrt(xc^2+yc^2)) > 1 && (abs(xc) > 0.2)
    if(sign(yc) == 1)
        if(sign(xc) == 1)
            psi = -acos(yc/sqrt(xc^2+yc^2))*180/pi;
            if(psi < -90)
                psi = -90;
            end
        else
            psi = acos(yc/sqrt(xc^2+yc^2))*180/pi;
            if(psi > 90)
                psi = 90;
            end
        end
    else
        if(sign(xc) == -1)
            psi = 90;
        else
            psi = -90;
        end
    end
else
    psi = 0;
end

== matlab function drone_simul10/Mapping d'un gamepad Xbox/Conversion X et Y/Deplacement élémentaire ==
  data: u input; y output
function y = Dd(u)

if u == 0
    y = [0;1];
elseif u == 45
    y = sqrt(2)/2*[1; 1];
elseif u == 90
    y = [1;0];
elseif u == 135
    y = sqrt(2)/2*[1;-1];
elseif u == 180
    y = [0;-1];
elseif u == 255
    y = sqrt(2)/2*[-1;-1];
elseif u == 270
    y = [-1;0];
elseif u == 315
    y = sqrt(2)/2*[-1;1];
else
    y = [0;0];
end

== matlab function drone_simul10/MATLAB Function ==
  data: Y input; X input; u1 output; Psi input; u2 output; u3 output; u4 output
function [u1, u2, u3, u4] = convertisseur(Y, X, Psi)


Comm = [sign(X), sign(Y),sign(Psi)];

Log = [0 1 1 0;
       1 1 0 0;
       0 1 0 1;
       1 0 0 1;
       0 0 1 1;
       1 0 1 0];

Prop = [0 0 0 0];

if Comm(1) == -1
    Prop = Prop + abs(X)*Log(4,:);
elseif Comm(1) == 1
    Prop = Prop + abs(X)*Log(1,:);
else
    Prop = Prop + [0 0 0 0];
end

if Comm(2) == -1
    Prop = Prop + abs(Y)*Log(5,:);
elseif Comm(2) == 1
    Prop = Prop + abs(Y)*Log(2,:);
else
    Prop = Prop + [0 0 0 0];
end

if Comm(3) == -1
    Prop = Prop + abs(Psi)*Log(6,:);
elseif Comm(3) == 1
    Prop = Prop + abs(Psi)*Log(3,:);
else
    Prop = Prop + [0 0 0 0];
end

Prop;

u1 = Prop(1);
u2 = Prop(2);
u3 = Prop(3);
u4 = Prop(4);

== matlab function drone_simul10/Mapping d'un gamepad Xbox/Conversion X et Y/Subsystem1/MATLAB Function2 ==
  data: u input; y output; c1 input; c2 input; b input; Condition input
function y = cas(u, c1, c2, b, Condition)

if ((u == b) && (Condition==655.35))
    y = c1;
else
    y = c2;
end

== matlab function drone_simul10/Mapping d'un gamepad Xbox/Conversion X et Y/Subsystem2/MATLAB Function2 ==
  data: u input; y output; c1 input; c2 input; b input; Condition input
function y = cas(u, c1, c2, b, Condition)

if ((u == b) && (Condition==655.35))
    y = c1;
else
    y = c2;
end

== matlab function drone_simul10/Mapping d'un gamepad Xbox/Subsystem3/MATLAB Function2 ==
  data: u input; y output; c1 input; c2 input; b input; Condition input
function y = cas(u, c1, c2, b, Condition)

if ((u == b) && (Condition==655.35))
    y = c1;
else
    y = c2;
end
